simulink model "MassSpringDamper"  (R2020b)
settings: Solver=VariableStepAuto  StartTime=0.0  StopTime=10.0  RelTol=1e-3
values from neighbouring files (symbols this model uses):
  b = 10    [MassSpringDamper_Integration.m]
  k = 20    [MassSpringDamper_Integration.m]
  Kd = 50    [MassSpringDamper_Integration.m]
  Ki = 300    [MassSpringDamper_Integration.m]
  Kp = 350    [MassSpringDamper_Integration.m]
  M = 1    [MassSpringDamper_Integration.m]
  Step_Value = 1    [MassSpringDamper_Integration.m]
settings Model: Creator=ApriZon  LastModifiedBy=ApriZon

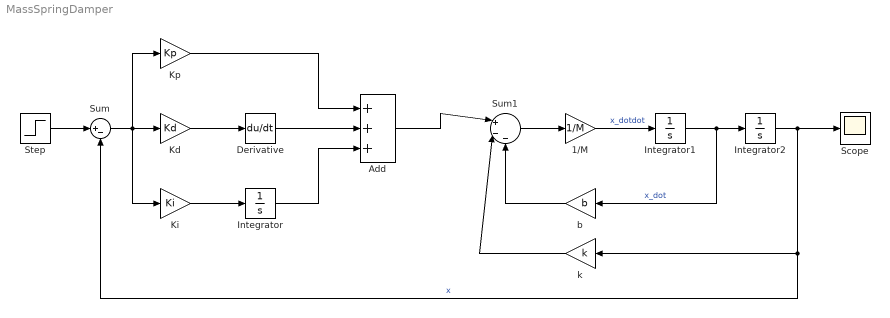
== system MassSpringDamper ==
  1/M : Gain  Gain=1/M
  Add : Sum  Inputs=+++
  Derivative : Derivative
  Integrator : Integrator
  Integrator1 : Integrator
  Integrator2 : Integrator
  Kd : Gain  Gain=Kd
  Ki : Gain  Gain=Ki
  Kp : Gain  Gain=Kp
  Scope : Scope
  Step : Step  After=Step_Value  SampleTime=0
  Sum : Sum  Inputs=|+-
  Sum1 : Sum  Inputs=|+--
  b : Gain  Gain=b
  k : Gain  Gain=k
  wires:
  Step/1 -> Sum/1
  Sum/1 -> Ki/1, Kp/1, Kd/1
  Kd/1 -> Derivative/1
  Ki/1 -> Integrator/1
  Derivative/1 -> Add/2
  Kp/1 -> Add/1
  Integrator/1 -> Add/3
  Add/1 -> Sum1/1
  k/1 -> Sum1/2
  b/1 -> Sum1/3
  Sum1/1 -> 1/M/1
  1/M/1 -> Integrator1/1  "x_dotdot"
  Integrator1/1 -> b/1, Integrator2/1  "x_dot"
  Integrator2/1 -> k/1, Sum/2, Scope/1  "x"
